simulink model "Bridge_simu_E0_test"  (R2022a)
settings: Solver=ode4  StartTime=t_init  StopTime=t_final  FixedStep=t_step  RelTol=1e-3
values from neighbouring files (symbols this model uses):
  As = [zeros(cant_modos) eye(cant_modos); -Me\Ke -Me\Ce]    [Bridge_model_E0.m]
  Bs = [zeros(cant_modos); Me\Ge]    [Bridge_model_E0.m]
  Cs = [eye(cant_modos) zeros(cant_modos) ; zeros(cant_modos) eye(cant_modos); -Me\Ke -Me\Ce]    [Bridge_model_E0.m]
  Ds = [zeros(cant_modos) ; zeros(cant_modos); Me\Ge]    [Bridge_model_E0.m]
settings Model: Creator=conni  LastModifiedBy=LEGION
settings DebuggingCC: UnconnectedInputMsg=warning  UnconnectedOutputMsg=warning  UnconnectedLineMsg=warning  SFMachineParentedDataDiag=warning
settings SFSimCC: CustomCodeUndefinedFunction=UseInterfaceOnly
settings RTWCC: DLArmComputeVersion=19.05

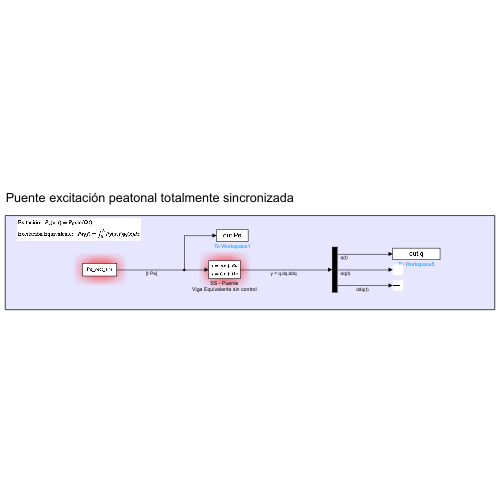
[thumbnail: Simulink's stored preview of the top-level diagram]
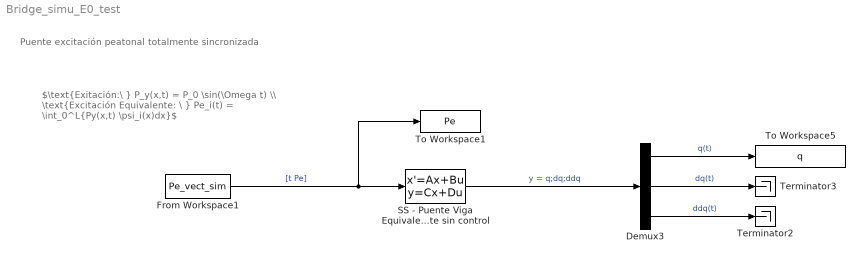
== system Bridge_simu_E0_test ==
  note: $\text{Exitación:\ } P_y(x,t) = P_0 \sin(\Omega t) \\ \text{Excitación Equivalente: \ } Pe_i(t) = \int_0^L{Py(x,t) \psi_i(x)dx}$
  note: Puente excitación peatonal totalmente sincronizada
  Demux3 : Demux  Outputs=3
  From Workspace1 : FromWorkspace  VariableName=Pe_vect_sim  OutputAfterFinalValue=Setting to zero
  SS - Puente Viga Equivalente sin control : StateSpace  A=As  B=Bs  C=Cs  D=Ds  InitialCondition=0
  Terminator2 : Terminator
  Terminator3 : Terminator
  To Workspace1 : ToWorkspace  VariableName=Pe  SaveFormat=Timeseries  SampleTime=-1
  To Workspace5 : ToWorkspace  VariableName=q  SaveFormat=Timeseries  SampleTime=-1
  wires:
  SS - Puente Viga Equivalente sin control/1 -> Demux3/1  "y = q;dq;ddq"
  Demux3/1 -> To Workspace5/1  "q(t)"
  Demux3/2 -> Terminator3/1  "dq(t)"
  Demux3/3 -> Terminator2/1  "ddq(t)"
  From Workspace1/1 -> To Workspace1/1, SS - Puente Viga Equivalente sin control/1  "[t Pe]"
